simulink library "motohawk_can_protocols_lib"  (Simulink 5.1)
libraries: MotoHawk_lib x24, simulink x4
settings Model: LastModifiedBy=Chris_Doyle  ProdHWDeviceType=Microprocessor

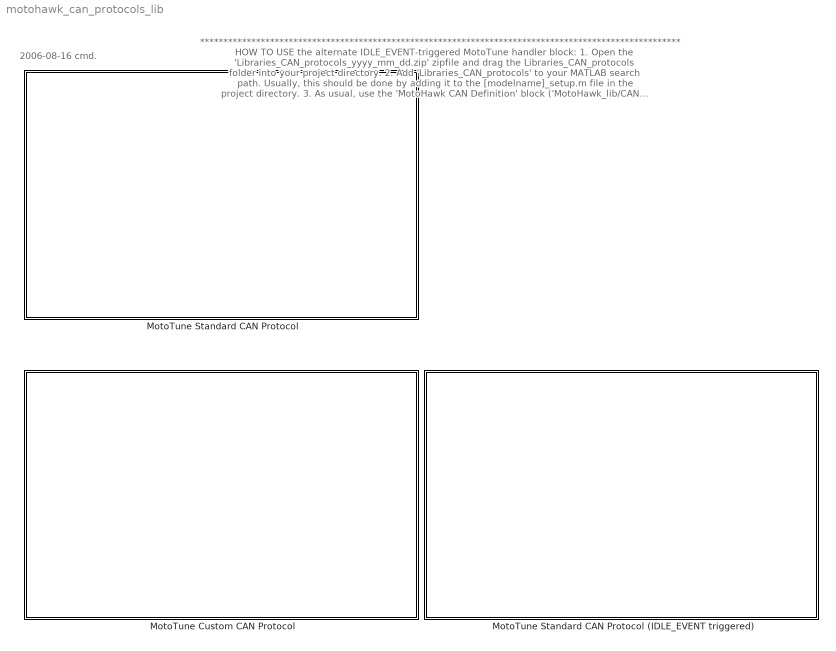
== system motohawk_can_protocols_lib ==
  note: 2006-08-16 cmd.
  note: *******************************************************************************************************
      | HOW TO USE the alternate IDLE_EVENT-triggered MotoTune handler block:
      | 1.  Open the 'Libraries_CAN_protocols_yyyy_mm_dd.zip' zipfile and drag the
      |      Libraries_CAN_protocols folder into your project directory.
      | 2.  Add 'Libraries_CAN_protocols' to your MATLAB search path.  Usually, this should
      |      be done by adding it to the [modelname]_setup.m file in the project directory.
      | 3.  As usual, use the 'MotoHawk CAN Definition' block ('MotoHawk_lib/CAN Blocks/
      |      CAN Definition') to define mask parameters for a CAN bus's bit timing and transmit
      |      queue size, but UN-check the 'Install MotoTune Protocol' checkbox.
      | 4.  At the MATLAB prompt, open the alternate-MotoTune-handler library by typing:
      |      >> motohawk_can_protocols_lib
      | 5.  Drag the IDLE_EVENT-triggered MotoTune handler block ('motohawk_can_
      |      protocols_lib/MotoTune Standard CAN Protocol (IDLE_EVENT triggered)') into
      |      your model and set its mask parameters appropriately.
      | 6.  Consume a beverage of your preference to celebrate your successful transition
      |      to the IDLE_EVENT-triggered MotoTune handler.
      | *******************************************************************************************************
      |                                                        _|   |_
      |                                                         \    /
      |                                                          \  /
      |                                                           \/
  MotoTune Custom CAN Protocol : Subsystem  mask(MotoTune CAN Protocol Handler){image_file='mototune.jpg', mtninstance='MotoTune1', channel=1, rxid=hex2dec('c02'), rxidtype=1, rxidmasknom=hex2dec('1fff00ff'), txid=hex2dec('020c'), txidtype=1, reprogcity=hex2dec('c')}
      mask prompts: image_file "imfileImage File"; mtninstance "MotoTune Handler Instance Name (unique string)"; channel "CAN Channel (integer)"; rxid "Receive ID"; rxidtype "Receive ID Type (0=Std, 1=Ext)"; rxidmasknom "Receive ID Mask"; txid "Transmit ID"; txidtype "Transmit ID Type (0=Std, 1=Ext)"; reprogcity "Reprogram City ID (uint8)"
      mask help:
      | Handle a MotoTune connection via CAN.
      |
      | MotoTune Handler Instance Name: A unique valid c name
      | that identifies this instance of a MotoTune connection.
      |
      | CAN Channel:  The hardware channel on which to make the
      | connection.
      |
      | Receive ID:  The nominal receive ID that MotoTune requests
      | will be received upon.
      |
      | Receive ID Type: Standard (11 bit) or Extended (29 bit) id.
      |
      | Receive ID Mask:  The bits of the Receive ID that must match.
      |
      | Transmit ID: The ID on which the module will reply to the
      | MotoTune request.
      |
      | Transmit ID Type: Standard (11 bit) or Extended (29 bit) id.
      |
      | ---------------------------------------------------------------------
      | Copyright 2005 MotoTron, Corp.  All Rights Reserved.
      mask init:
      | try,
      | 	img = imread(image_file);
      | 	motohawk_block_image(gcb, image_file);
      | catch,
      | 	img = imread('image_not_found.jpg');
      | end
      | 
      | e = {'(std)','(ext)'};
      | reqbits = hex2dec('1f00ffff'); 
      | rxidmask = bitand(uint32(rxidmasknom),uint32(reqbits));
      | rxlbl = sprintf('\\fontname{courier new}Chan  : CAN\\_%g\\newlineRx ID : 0x%08x %s\\newlineID Adj: 0x%08x', channel,rxid,e{rxidtype+1},double(bitxor(uint32(rxidmask),uint32(reqbits))));
      | txlbl = sprintf('\\fontname{courier new}Chan  : CAN\\_%g\\newlineTx ID : 0x%08x %s\\newlineProg City ID: 0x%02x', channel,txid,e{txidtype+1},double(uint8(reprogcity)));
      settings: MoveFcn=motohawk_block_image(gcb, motohawk_get_param_ws(gcb, 'image_file'));
      mask Display:
      | patch([0 0 1 1], [0 0.075 0.075 0], [230/255 0/255 0/255])
      | patch([0 0 1 1], [0.025 0.05 0.05 0.025], [150/255 0/255 0/255])
      | patch([0 0 1 1], [0 0.025 0.025 0], [0/255 0/255 0/255])
      | image(img,[0 0.25 0.75 0.75]);
      | 
      | text(0.99,0.57,['\fontname{Arial}\fontsize{18}\bfMotoTune Handler\fontsize{12}\newline\rmInstance: ' strrep(mtninstance,'_','\_')],'texmode','on','HorizontalAlignment','Right')
      | 
      | text(0.01,0.22,['\fontname{Arial}\fontsize{18}\bfRx\fontsize{12}\newline\rm' rxlbl],'texmode','on','HorizontalAlignment','Left')
      | text(0.99,0.22,['\fontname{Arial}\fontsize{18}\bfTx\fontsize{12}\newline\rm' txlbl],'texmode','on','HorizontalAlignment','Right')
  MotoTune Standard CAN Protocol : Subsystem  mask(MotoTune CAN Protocol Handler){image_file='mototune.jpg', mtninstance='CAN_1', channel=1, reprogcity=hex2dec('b')}
      mask prompts: image_file "imfileImage File"; mtninstance "MotoTune Handler Instance Name (unique string)"; channel "CAN Channel (integer)"; reprogcity "Default City ID (uint8)"
      mask help:
      | Handle a MotoTune connection via CAN.
      |
      | MotoTune Handler Instance Name: A unique valid c name
      | that identifies this instance of a MotoTune connection. For
      | standard operation use 'CAN_1' or 'CAN_2'
      |
      | CAN Channel:  The hardware channel on which to make the
      | connection.
      |
      | City ID: The Smartcraft City ID that identifies this module.
      | 0x0b = PCM-1
      | 0x0c = PCM-2
      | 0x91 = uCHI-1
      | 0x92 = uCHI-2
      |
      | ---------------------------------------------------------------------
      | Copyright 2005 MotoTron, Corp.  All Rights Reserved.
      mask init:
      | try,
      | 	img = imread(image_file);
      | 	motohawk_block_image(gcb, image_file);
      | catch,
      | 	img = imread('image_not_found.jpg');
      | end
      | 
      | e = {'(std)','(ext)'};
      | reqbits = hex2dec('1f00ffff'); 
      | citylbl = sprintf('City ID: 0x%02x', double(uint8(reprogcity)));
      | chlbl = sprintf('Ch: CAN\\_%g', double(uint8(channel)));
      settings: MoveFcn=motohawk_block_image(gcb, motohawk_get_param_ws(gcb, 'image_file'));
      mask Display:
      | patch([0 0 1 1], [0 0.075 0.075 0], [230/255 0/255 0/255])
      | patch([0 0 1 1], [0.025 0.05 0.05 0.025], [150/255 0/255 0/255])
      | patch([0 0 1 1], [0 0.025 0.025 0], [0/255 0/255 0/255])
      | image(img,[0 0.25 0.75 0.75]);
      | 
      | text(0.99,0.50,['\fontname{Arial}\fontsize{18}\bfMotoTune Handler\fontsize{12}\newline\rmInstance: ' strrep(mtninstance,'_','\_') '\newline' citylbl '\newline' chlbl],'texmode','on','HorizontalAlignment','Right')
  MotoTune Standard CAN Protocol (IDLE_EVENT triggered) : Subsystem  mask(MotoTune CAN Protocol Handler){image_file='mototune.jpg', mtninstance='CAN_1', channel=1, reprogcity=hex2dec('b')}
      mask prompts: image_file "imfileImage File"; mtninstance "MotoTune Handler Instance Name (unique string)"; channel "CAN Channel (integer)"; reprogcity "Default City ID (uint8)"
      mask help:
      | Handle a MotoTune connection via CAN.
      |
      | MotoTune Handler Instance Name: A unique valid c name
      | that identifies this instance of a MotoTune connection. For
      | standard operation use 'CAN_1' or 'CAN_2'
      |
      | CAN Channel:  The hardware channel on which to make the
      | connection.
      |
      | City ID: The Smartcraft City ID that identifies this module.
      | 0x0b = PCM-1
      | 0x0c = PCM-2
      | 0x91 = uCHI-1
      | 0x92 = uCHI-2
      |
      | ---------------------------------------------------------------------
      | Copyright 2005 MotoTron, Corp.  All Rights Reserved.
      mask init: same as motohawk_can_protocols_lib/MotoTune Standard CAN Protocol
      settings: MoveFcn=motohawk_block_image(gcb, motohawk_get_param_ws(gcb, 'image_file'));
      mask Display:
      | patch([0 0 1 1], [0 0.075 0.075 0], [230/255 0/255 0/255])
      | patch([0 0 1 1], [0.025 0.05 0.05 0.025], [150/255 0/255 0/255])
      | patch([0 0 1 1], [0 0.025 0.025 0], [0/255 0/255 0/255])
      | image(img,[0 0.25 0.75 0.75]);
      | 
      | text(0.99,0.50,['\fontname{Arial}\fontsize{18}\bfMotoTune Handler\fontsize{12}\newline\rmInstance: ' strrep(mtninstance,'_','\_') '\newline' citylbl '\newline' chlbl '\newlineIDLE\_EVENT triggered'],'texmode','on','HorizontalAlignment','Right')

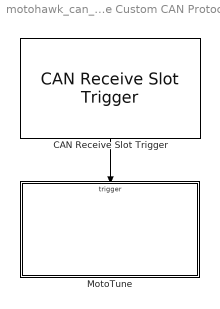
== system motohawk_can_protocols_lib/MotoTune Custom CAN Protocol ==
  CAN Receive Slot Trigger : MotoHawk_lib/CAN Blocks/CAN Receive Slot Trigger  Tag=Trigger  Orientation=down  slot=mtninstance  inherited=on
  MotoTune : Subsystem
  wires:
  CAN Receive Slot Trigger/1 -> MotoTune/Trigger

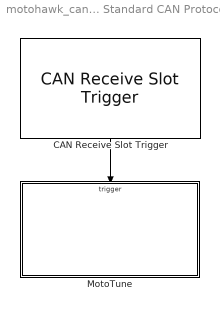
== system motohawk_can_protocols_lib/MotoTune Standard CAN Protocol ==
  CAN Receive Slot Trigger : MotoHawk_lib/CAN Blocks/CAN Receive Slot Trigger  Tag=Trigger  Orientation=down  slot=mtninstance  inherited=on
  MotoTune : Subsystem
  wires:
  CAN Receive Slot Trigger/1 -> MotoTune/Trigger

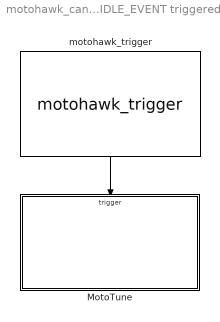
== system motohawk_can_protocols_lib/MotoTune Standard CAN Protocol (IDLE_EVENT triggered) ==
  MotoTune : Subsystem
  motohawk_trigger : MotoHawk_lib/Trigger Blocks/motohawk_trigger  Tag=Trigger  Orientation=down  trigger=IDLE_EVENT  priority_order=0  inherited=on  run_disabled=on  override_app_monitor=on  target=All
  wires:
  motohawk_trigger/1 -> MotoTune/Trigger

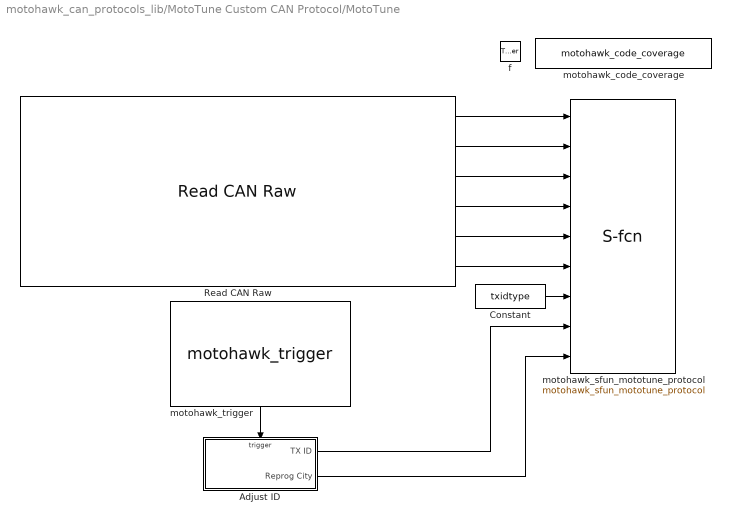
== system motohawk_can_protocols_lib/MotoTune Custom CAN Protocol/MotoTune ==
  f : TriggerPort  TriggerType=function-call
  Adjust ID : Subsystem
  Constant : Constant  Value=txidtype  ShowAdditionalParam=on
  Read CAN Raw : MotoHawk_lib/CAN Blocks/Read CAN Raw  bus=channel  id_ext=1  id=double(rxid)  id_mask=double(rxidmask)  pay=[]  pay_mask=[]  queue=4  slot=mtninstance  valid=on  stale=on
  motohawk_code_coverage : MotoHawk_lib/Extra Development Blocks/motohawk_code_coverage
  motohawk_sfun_mototune_protocol : S-Function  FunctionName=motohawk_sfun_mototune_protocol  Parameters=uint8(ch)  mask(MotoTune Control Core Interface){ch=channel}
      mask prompts: ch "CAN Channel"
      mask help:
      | Interface to Control Core MotoTune handler.
      |
      | ---------------------------------------------------------------------
      | Copyright 2005 MotoTron, Corp.  All Rights Reserved.
      mask init:
      | lbl = 'MotoTune';
      mask Display:
      | patch([0 0 1 1], [0 1 1 0], [220/255 220/255 220/255]);
      | patch([0 0 1 1], 0.5*[0 0.075 0.075 0], [230/255 0/255 0/255]);
      | patch([0 0 1 1], 0.5*[0.025 0.05 0.05 0.025], [150/255 0/255 0/255]);
      | patch([0 0 1 1], 0.5*[0 0.025 0.025 0], [0/255 0/255 0/255]);
      | text(0.5, 0.85, lbl, 'texmode','on','VerticalAlignment','Top','HorizontalAlignment','Center');
  motohawk_trigger : MotoHawk_lib/Trigger Blocks/motohawk_trigger  Tag=Trigger  Orientation=down  trigger=STARTUP_EVENT  priority_order=0  inherited=on  run_disabled=off  override_app_monitor=off  target=ECU555_80
  wires:
  Adjust ID/2(Reprog City) -> motohawk_sfun_mototune_protocol/9
  motohawk_trigger/1 -> Adjust ID/Trigger
  Constant/1 -> motohawk_sfun_mototune_protocol/7
  Adjust ID/1(TX ID) -> motohawk_sfun_mototune_protocol/8
  Read CAN Raw/6 -> motohawk_sfun_mototune_protocol/6
  Read CAN Raw/5 -> motohawk_sfun_mototune_protocol/5
  Read CAN Raw/4 -> motohawk_sfun_mototune_protocol/4
  Read CAN Raw/3 -> motohawk_sfun_mototune_protocol/3
  Read CAN Raw/2 -> motohawk_sfun_mototune_protocol/2
  Read CAN Raw/1 -> motohawk_sfun_mototune_protocol/1

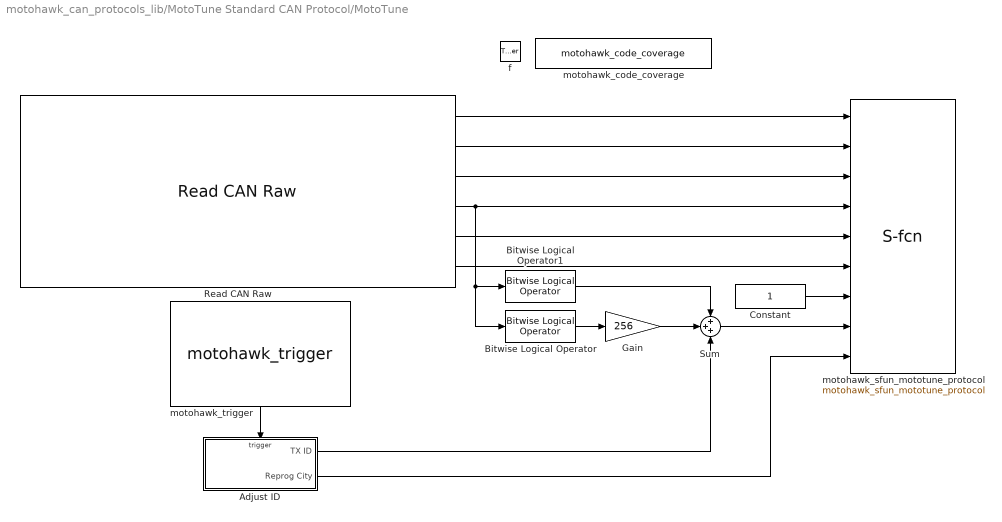
== system motohawk_can_protocols_lib/MotoTune Standard CAN Protocol/MotoTune ==
  f : TriggerPort  TriggerType=function-call
  Adjust ID : Subsystem
  Bitwise Logical Operator : simulink/Math Operations/Bitwise Logical Operator  Operator=AND  Operand2='000000FF'
  Bitwise Logical Operator1 : simulink/Math Operations/Bitwise Logical Operator  Operator=AND  Operand2='1FFF0000'
  Constant : Constant  ShowAdditionalParam=on
  Gain : Gain  Gain=256  SaturateOnIntegerOverflow=on
  Read CAN Raw : MotoHawk_lib/CAN Blocks/Read CAN Raw  bus=channel  id_ext=1  id=double(reprogcity*256+2)  id_mask=double(hex2dec('000000f0'))  pay=[]  pay_mask=[]  queue=4  slot=mtninstance  valid=on  stale=on
  Sum : Sum  Inputs=+++  SaturateOnIntegerOverflow=on
  motohawk_code_coverage : MotoHawk_lib/Extra Development Blocks/motohawk_code_coverage
  motohawk_sfun_mototune_protocol : S-Function  FunctionName=motohawk_sfun_mototune_protocol  Parameters=uint8(ch)  mask(MotoTune Control Core Interface){ch=channel}
      mask prompts: ch "CAN Channel"
      mask help:
      | Interface to Control Core MotoTune handler.
      |
      | ---------------------------------------------------------------------
      | Copyright 2005 MotoTron, Corp.  All Rights Reserved.
      mask init:
      | lbl = 'MotoTune';
      mask Display:
      | patch([0 0 1 1], [0 1 1 0], [220/255 220/255 220/255]);
      | patch([0 0 1 1], 0.5*[0 0.075 0.075 0], [230/255 0/255 0/255]);
      | patch([0 0 1 1], 0.5*[0.025 0.05 0.05 0.025], [150/255 0/255 0/255]);
      | patch([0 0 1 1], 0.5*[0 0.025 0.025 0], [0/255 0/255 0/255]);
      | text(0.5, 0.85, lbl, 'texmode','on','VerticalAlignment','Top','HorizontalAlignment','Center');
  motohawk_trigger : MotoHawk_lib/Trigger Blocks/motohawk_trigger  Tag=Trigger  Orientation=down  trigger=STARTUP_EVENT  priority_order=0  inherited=on  run_disabled=off  override_app_monitor=off  target=ECU555_80
  wires:
  Sum/1 -> motohawk_sfun_mototune_protocol/8
  Bitwise Logical Operator1/1 -> Sum/1
  Gain/1 -> Sum/2
  Adjust ID/1(TX ID) -> Sum/3
  Bitwise Logical Operator/1 -> Gain/1
  Read CAN Raw/1 -> motohawk_sfun_mototune_protocol/1
  Read CAN Raw/2 -> motohawk_sfun_mototune_protocol/2
  Read CAN Raw/3 -> motohawk_sfun_mototune_protocol/3
  Read CAN Raw/4 -> Bitwise Logical Operator1/1, Bitwise Logical Operator/1, motohawk_sfun_mototune_protocol/4
  Read CAN Raw/5 -> motohawk_sfun_mototune_protocol/5
  Read CAN Raw/6 -> motohawk_sfun_mototune_protocol/6
  Constant/1 -> motohawk_sfun_mototune_protocol/7
  motohawk_trigger/1 -> Adjust ID/Trigger
  Adjust ID/2(Reprog City) -> motohawk_sfun_mototune_protocol/9

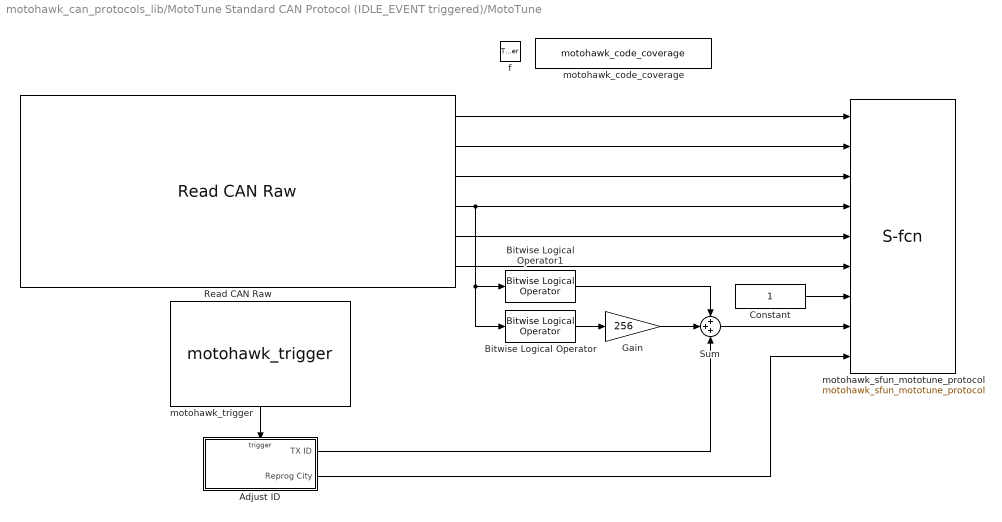
== system motohawk_can_protocols_lib/MotoTune Standard CAN Protocol (IDLE_EVENT triggered)/MotoTune ==
  f : TriggerPort  TriggerType=function-call
  Adjust ID : Subsystem
  Bitwise Logical Operator : simulink/Math Operations/Bitwise Logical Operator  Operator=AND  Operand2='000000FF'
  Bitwise Logical Operator1 : simulink/Math Operations/Bitwise Logical Operator  Operator=AND  Operand2='1FFF0000'
  Constant : Constant  ShowAdditionalParam=on
  Gain : Gain  Gain=256  SaturateOnIntegerOverflow=on
  Read CAN Raw : MotoHawk_lib/CAN Blocks/Read CAN Raw  bus=channel  id_ext=1  id=double(reprogcity*256+2)  id_mask=double(hex2dec('00000000'))  pay=[]  pay_mask=[]  queue=4  slot=mtninstance  valid=on  stale=on
  Sum : Sum  Inputs=+++  SaturateOnIntegerOverflow=on
  motohawk_code_coverage : MotoHawk_lib/Extra Development Blocks/motohawk_code_coverage
  motohawk_sfun_mototune_protocol : S-Function  FunctionName=motohawk_sfun_mototune_protocol  Parameters=uint8(ch)  mask(MotoTune Control Core Interface){ch=channel}
      mask prompts: ch "CAN Channel"
      mask help:
      | Interface to Control Core MotoTune handler.
      |
      | ---------------------------------------------------------------------
      | Copyright 2005 MotoTron, Corp.  All Rights Reserved.
      mask init:
      | lbl = 'MotoTune';
      mask Display:
      | patch([0 0 1 1], [0 1 1 0], [220/255 220/255 220/255]);
      | patch([0 0 1 1], 0.5*[0 0.075 0.075 0], [230/255 0/255 0/255]);
      | patch([0 0 1 1], 0.5*[0.025 0.05 0.05 0.025], [150/255 0/255 0/255]);
      | patch([0 0 1 1], 0.5*[0 0.025 0.025 0], [0/255 0/255 0/255]);
      | text(0.5, 0.85, lbl, 'texmode','on','VerticalAlignment','Top','HorizontalAlignment','Center');
  motohawk_trigger : MotoHawk_lib/Trigger Blocks/motohawk_trigger  Tag=Trigger  Orientation=down  trigger=STARTUP_EVENT  priority_order=0  inherited=on  run_disabled=off  override_app_monitor=off  target=ECU555_80
  wires:
  Sum/1 -> motohawk_sfun_mototune_protocol/8
  Bitwise Logical Operator1/1 -> Sum/1
  Gain/1 -> Sum/2
  Adjust ID/1(TX ID) -> Sum/3
  Bitwise Logical Operator/1 -> Gain/1
  Read CAN Raw/1 -> motohawk_sfun_mototune_protocol/1
  Read CAN Raw/2 -> motohawk_sfun_mototune_protocol/2
  Read CAN Raw/3 -> motohawk_sfun_mototune_protocol/3
  Read CAN Raw/4 -> Bitwise Logical Operator1/1, Bitwise Logical Operator/1, motohawk_sfun_mototune_protocol/4
  Read CAN Raw/5 -> motohawk_sfun_mototune_protocol/5
  Read CAN Raw/6 -> motohawk_sfun_mototune_protocol/6
  Constant/1 -> motohawk_sfun_mototune_protocol/7
  motohawk_trigger/1 -> Adjust ID/Trigger
  Adjust ID/2(Reprog City) -> motohawk_sfun_mototune_protocol/9

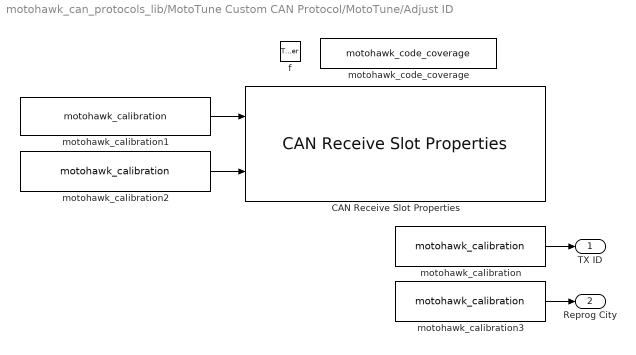
== system motohawk_can_protocols_lib/MotoTune Custom CAN Protocol/MotoTune/Adjust ID ==
  f : TriggerPort  TriggerType=function-call
  CAN Receive Slot Properties : MotoHawk_lib/CAN Blocks/CAN Receive Slot Properties  slot=mtninstance  id_filt=on  pay_filt=off
  motohawk_calibration : MotoHawk_lib/Calibration & Probing Blocks/motohawk_calibration  nam=[mtninstance 'TxID']  val=txid  storage=Calibration NV  show_more=on  name_source=Use Parameter  data_type=Inherit via back propagation  read_level=1  write_level=1  ovr_cals=on  view_as=Number  enum_struct={'Disabled', 'Enabled'}  use_help_units=on  help=['Transmit CAN ID for handler: ' mtninstance]  units=''  use_min_max=off  min_val=-inf  max_val=inf  use_precision=off  precision=''  gain=1  offset=0  exp=1  use_mototune_group=on  mototune_group=['MotoTune | ' mtninstance]
  motohawk_calibration1 : MotoHawk_lib/Calibration & Probing Blocks/motohawk_calibration  nam=[mtninstance 'RxID']  val=rxid  storage=Calibration NV  show_more=on  name_source=Use Parameter  data_type=Inherit via back propagation  read_level=1  write_level=1  ovr_cals=on  view_as=Number  enum_struct={'Disabled', 'Enabled'}  use_help_units=on  help=['Receive CAN ID for handler: ' mtninstance]  units=''  use_min_max=off  min_val=-inf  max_val=inf  use_precision=off  precision=''  gain=1  offset=0  exp=1  use_mototune_group=on  mototune_group=['MotoTune | ' mtninstance]
  motohawk_calibration2 : MotoHawk_lib/Calibration & Probing Blocks/motohawk_calibration  nam=[mtninstance 'RxIDMask']  val=bitxor(uint32(rxidmask),uint32(reqbits))  storage=Calibration NV  show_more=on  name_source=Use Parameter  data_type=Inherit via back propagation  read_level=1  write_level=1  ovr_cals=on  view_as=Number  enum_struct={'Disabled', 'Enabled'}  use_help_units=on  help=['Receive CAN ID Mask for handler: ' mtninstance]  units=''  use_min_max=off  min_val=-inf  max_val=inf  use_precision=off  precision=''  gain=1  offset=0  exp=1  use_mototune_group=on  mototune_group=['MotoTune | ' mtninstance]
  motohawk_calibration3 : MotoHawk_lib/Calibration & Probing Blocks/motohawk_calibration  nam=[mtninstance 'ReProgCityID']  val=reprogcity  storage=Calibration NV  show_more=on  name_source=Use Parameter  data_type=Inherit via back propagation  read_level=1  write_level=1  ovr_cals=on  view_as=Number  enum_struct={'Disabled', 'Enabled'}  use_help_units=on  help=['Reprogramming City ID for handler: ' mtninstance]  units=''  use_min_max=off  min_val=-inf  max_val=inf  use_precision=off  precision=''  gain=1  offset=0  exp=1  use_mototune_group=on  mototune_group=['MotoTune | ' mtninstance]
  motohawk_code_coverage : MotoHawk_lib/Extra Development Blocks/motohawk_code_coverage
  TX ID : Outport
  Reprog City : Outport  Port=2
  wires:
  motohawk_calibration3/1 -> Reprog City/1
  motohawk_calibration/1 -> TX ID/1
  motohawk_calibration2/1 -> CAN Receive Slot Properties/2
  motohawk_calibration1/1 -> CAN Receive Slot Properties/1

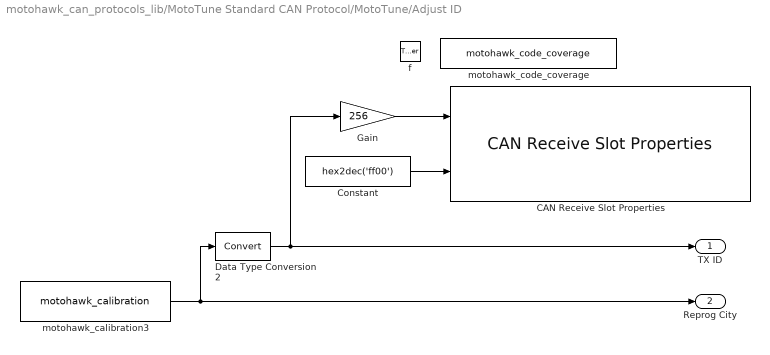
== system motohawk_can_protocols_lib/MotoTune Standard CAN Protocol/MotoTune/Adjust ID ==
  f : TriggerPort  TriggerType=function-call
  CAN Receive Slot Properties : MotoHawk_lib/CAN Blocks/CAN Receive Slot Properties  slot=mtninstance  id_filt=on  pay_filt=off
  Constant : Constant  Value=hex2dec('ff00')  ShowAdditionalParam=on
  Data Type Conversion2 : DataTypeConversion  DataType=uint32  SaturateOnIntegerOverflow=on
  Gain : Gain  Gain=256  SaturateOnIntegerOverflow=on
  motohawk_calibration3 : MotoHawk_lib/Calibration & Probing Blocks/motohawk_calibration  nam=['CityID_' mtninstance]  val=reprogcity  storage=Calibration NV  show_more=on  name_source=Use Parameter  data_type=uint8  read_level=1  write_level=1  ovr_cals=on  view_as=Number  enum_struct={'Disabled', 'Enabled'}  vector_style=Wide Row  use_help_units=on  help=['Reprogramming City ID for handler: ' mtninstance]  units=''  use_header_enum=off  row_header_enum={}  col_header_enum={}  use_min_max=off  min_val=-inf  max_val=inf  use_precision=off  precision=''  gain=1  offset=0  exp=1  use_mototune_group=on  mototune_group=['MotoTune | ' mtninstance]
  motohawk_code_coverage : MotoHawk_lib/Extra Development Blocks/motohawk_code_coverage
  TX ID : Outport
  Reprog City : Outport  Port=2
  wires:
  Data Type Conversion2/1 -> TX ID/1, Gain/1
  Constant/1 -> CAN Receive Slot Properties/2
  Gain/1 -> CAN Receive Slot Properties/1
  motohawk_calibration3/1 -> Reprog City/1, Data Type Conversion2/1

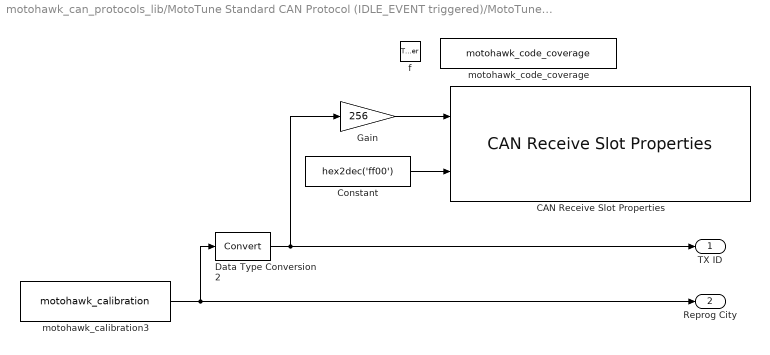
== system motohawk_can_protocols_lib/MotoTune Standard CAN Protocol (IDLE_EVENT triggered)/MotoTune/Adjust ID ==
  f : TriggerPort  TriggerType=function-call
  CAN Receive Slot Properties : MotoHawk_lib/CAN Blocks/CAN Receive Slot Properties  slot=mtninstance  id_filt=on  pay_filt=off
  Constant : Constant  Value=hex2dec('ff00')  ShowAdditionalParam=on
  Data Type Conversion2 : DataTypeConversion  DataType=uint32  SaturateOnIntegerOverflow=on
  Gain : Gain  Gain=256  SaturateOnIntegerOverflow=on
  motohawk_calibration3 : MotoHawk_lib/Calibration & Probing Blocks/motohawk_calibration  nam=['CityID_' mtninstance]  val=reprogcity  storage=Calibration NV  show_more=on  name_source=Use Parameter  data_type=uint8  read_level=1  write_level=1  ovr_cals=on  view_as=Number  enum_struct={'Disabled', 'Enabled'}  use_help_units=on  help=['Reprogramming City ID for handler: ' mtninstance]  units=''  use_min_max=off  min_val=-inf  max_val=inf  use_precision=off  precision=''  gain=1  offset=0  exp=1  use_mototune_group=on  mototune_group=['MotoTune | ' mtninstance]
  motohawk_code_coverage : MotoHawk_lib/Extra Development Blocks/motohawk_code_coverage
  TX ID : Outport
  Reprog City : Outport  Port=2
  wires:
  Data Type Conversion2/1 -> TX ID/1, Gain/1
  Constant/1 -> CAN Receive Slot Properties/2
  Gain/1 -> CAN Receive Slot Properties/1
  motohawk_calibration3/1 -> Reprog City/1, Data Type Conversion2/1
